simulink model "LV_Greensite"  (R2019b)
settings: Solver=ode4  StartTime=0.0  StopTime=140  FixedStep=0.01  RelTol=1e-3
values from neighbouring files (symbols this model uses):
  drywind =     [drywind.mat]
undefined symbols (not defined in the file or in its folder): GreensiteLPV, K, Qmax
libraries: cstblocks x6, simulink_extras x4, simulink x2
settings Model: SimulationMode=accelerator  Creator=Damhlaic  LastModifiedBy=mimmo
settings DataIOCC: ReturnWorkspaceOutputs=off
settings DebuggingCC: ArithmeticOperatorsInVariantConditions=warning
settings SFSimCC: CustomCodeUndefinedFunction=UseInterfaceOnly
settings RTWCC: TargetLang=C++
settings GRTTargetCC: TargetLangStandard=C++03 (ISO)  MultiInstanceERTCode=on  CodeInterfacePackaging=C++ class

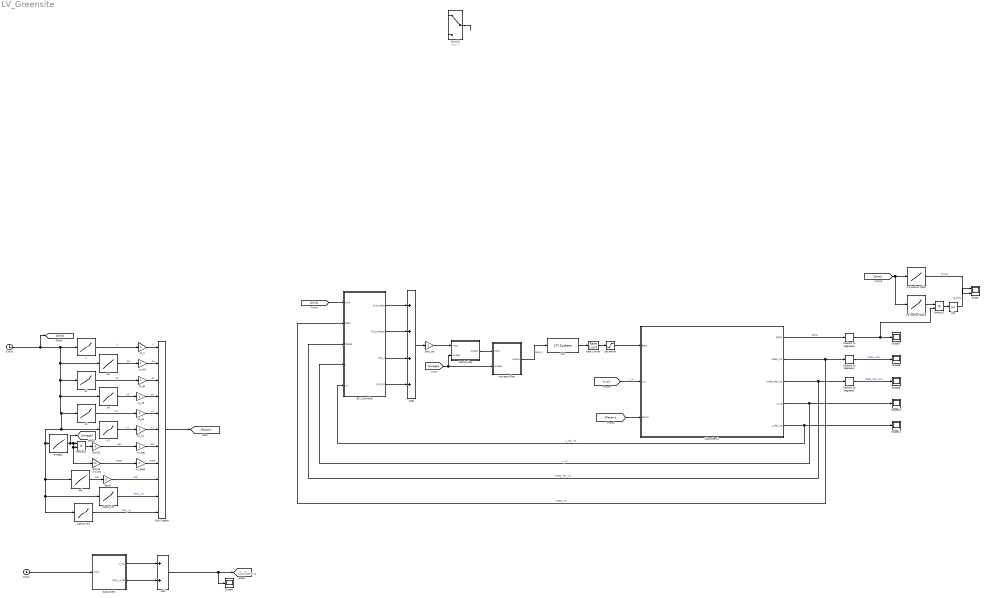
== system LV_Greensite ==
  note: 1445
      | 22360
      | 0.25
  1-D Lookup Table : Lookup_n-D  NumberOfTableDimensions=1  BreakpointsForDimension1=Qmax.time  Table=Qmax.Qalpha  InternalRulePriority=Speed  RndMeth=Simplest  InputSameDT=on
  1-D Lookup Table1 : Lookup_n-D  NumberOfTableDimensions=1  BreakpointsForDimension1=GreensiteLPV.Q.time  Table=GreensiteLPV.Q.Data  InternalRulePriority=Speed  RndMeth=Simplest  InputSameDT=on
  A6 : Lookup_n-D  NumberOfTableDimensions=1  BreakpointsForDimension1=GreensiteLPV.A6.Time  Table=GreensiteLPV.A6.Data  InternalRulePriority=Speed  RndMeth=Simplest  InputSameDT=on
  Abs : Abs
  Add : Sum
  Add1 : Sum  Inputs=++++
  BC_Controller : Subsystem
  Bus Creator : BusCreator  Inputs=11
  Clock : Clock
  Clock1 : Clock
  Gain12 : Gain  Gain=-1
  Gain13 : Gain  Gain=-2*0.005
  Gain5 : Gain  Gain=-1
  Gain_tot : Gain  Gain=-1
  K1 : Lookup_n-D  NumberOfTableDimensions=1  BreakpointsForDimension1=GreensiteLPV.K1.Time  Table=GreensiteLPV.K1.Data  InternalRulePriority=Speed  RndMeth=Simplest  InputSameDT=on
  Notch-Filter : Subsystem
  Product1 : Product
  Product2 : Product
  Radians to Degrees3 : simulink_extras/Transformations/Radians to Degrees
  Radians to Degrees4 : simulink_extras/Transformations/Radians to Degrees
  Radians to Degrees5 : simulink_extras/Transformations/Radians to Degrees
  Rate Limiter : RateLimiter  RisingSlewLimit=deg2rad(10)  FallingSlewLimit=-deg2rad(10)  SampleTimeMode=inherited
  Saturation : Saturate  UpperLimit=deg2rad(6)  LowerLimit=-deg2rad(6)
  Scope : Scope  NumInputPorts=2
  Scope{4,7..11} (6 alike) : Scope
  Subsystem : Subsystem
  Subsystem1 : Subsystem
  Switch2 : Switch  Criteria=u2 > Threshold  Threshold=7
  TVC : cstblocks/LTI System  sys=TVC_dyn  IC=[]
  V : Lookup_n-D  NumberOfTableDimensions=1  BreakpointsForDimension1=GreensiteLPV.V.Time  Table=GreensiteLPV.V.Data  InternalRulePriority=Speed  RndMeth=Simplest  InputSameDT=on
  a1 : Lookup_n-D  NumberOfTableDimensions=1  BreakpointsForDimension1=GreensiteLPV.a1.Time  Table=GreensiteLPV.a1.Data  InternalRulePriority=Speed  RndMeth=Simplest  InputSameDT=on
  a3 : Lookup_n-D  NumberOfTableDimensions=1  BreakpointsForDimension1=GreensiteLPV.a3.Time  Table=GreensiteLPV.a3.Data  InternalRulePriority=Speed  RndMeth=Simplest  InputSameDT=on
  a4 : Lookup_n-D  NumberOfTableDimensions=1  BreakpointsForDimension1=GreensiteLPV.a4.Time  Table=GreensiteLPV.a4.Data  InternalRulePriority=Speed  RndMeth=Simplest  InputSameDT=on
  aqk : Lookup_n-D  NumberOfTableDimensions=1  BreakpointsForDimension1=GreensiteLPV.aqk.Time  Table=GreensiteLPV.aqk.Data  InternalRulePriority=Speed  RndMeth=Simplest  InputSameDT=on
  low-pass filter : Subsystem
  omega1 : Lookup_n-D  NumberOfTableDimensions=1  BreakpointsForDimension1=GreensiteLPV.omega.Time  Table=GreensiteLPV.omega.Data  InternalRulePriority=Speed  RndMeth=Simplest  InputSameDT=on
  sigma_ins : Lookup_n-D  NumberOfTableDimensions=1  BreakpointsForDimension1=GreensiteLPV.sigma_ins.Time  Table=GreensiteLPV.sigma_ins.Data  InternalRulePriority=Speed  RndMeth=Simplest  InputSameDT=on
  sigma_ins1 : Lookup_n-D  NumberOfTableDimensions=1  BreakpointsForDimension1=GreensiteLPV.phi_ins.Time  Table=GreensiteLPV.phi_ins.Data  InternalRulePriority=Speed  RndMeth=Simplest  InputSameDT=on
  un_A6 : Gain
  un_K1 : Gain
  un_V : Gain
  un_a1 : Gain
  un_a3 : Gain
  un_a4 : Gain
  un_aqq : Gain
  un_aqqd : Gain
  wires:
  V/1 -> un_V/1  "V"
  A6/1 -> un_A6/1  "A6"
  a1/1 -> un_a1/1  "a1"
  a3/1 -> un_a3/1  "a3"
  a4/1 -> un_a4/1  "a4"
  Gain12/1 -> un_aqq/1  "aqq"
  Gain13/1 -> un_aqqd/1  "aqqd"
  aqk/1 -> Gain5/1  "aqk"
  sigma_ins/1 -> Bus Creator/10  "RMC_ins"
  Bus Creator/1 -> [Param]
  K1/1 -> un_K1/1  "K1"
  BC_Controller/4("Out_zd ") -> Add1/4
  BC_Controller/3(Out_z) -> Add1/3
  Radians to Degrees3/1 -> Scope9/1  "theta_dot_AAC"
  low-pass filter/1(output) -> TVC/1  "beta_c"
  Subsystem1/1(alpha) -> Radians to Degrees5/1  "alpha"
  [v_w] -> Subsystem1/2(v_w)  "v_w"
  Subsystem1/5(z_dot_ins) -> BC_Controller/5(zd), Scope11/1  "z_dot_ins"
  Subsystem1/4(z_ins) -> BC_Controller/4(z), Scope10/1  "z_ins"
  Subsystem1/3(theta_dot_ins) -> BC_Controller/3(thetad), Radians to Degrees3/1  "theta_dot_ins"
  BC_Controller/2(Out_thetad) -> Add1/2
  BC_Controller/1(Out_theta) -> Add1/1
  Add1/1 -> Gain_tot/1
  [Param] -> Subsystem1/3(param)
  Subsystem1/2(theta_ins) -> Radians to Degrees4/1, BC_Controller/2(theta)  "theta_ins"
  un_A6/1 -> Bus Creator/2  "A6"
  un_K1/1 -> Bus Creator/6  "K1"
  un_aqqd/1 -> Bus Creator/8  "aqqd"
  un_aqq/1 -> Bus Creator/7  "aqq"
  sigma_ins1/1 -> Bus Creator/11  "TMC_ins"
  Clock1/1 -> omega1/1, sigma_ins1/1, sigma_ins/1, aqk/1, K1/1, a4/1, a3/1, a1/1, A6/1, V/1, [time]
  Radians to Degrees5/1 -> Product2/2, Scope7/1
  un_V/1 -> Bus Creator/1  "V"
  un_a1/1 -> Bus Creator/3  "a1"
  un_a3/1 -> Bus Creator/4  "a3"
  un_a4/1 -> Bus Creator/5  "a4"
  Subsystem/2(noisy_wind) -> Add/2
  Subsystem/1(v_wp) -> Add/1
  Product1/1 -> Gain12/1
  [time] -> BC_Controller/1(time)
  Gain5/1 -> Bus Creator/9  "aqk"
  1-D Lookup Table1/1 -> Product2/1
  Product2/1 -> Abs/1
  1-D Lookup Table/1 -> Scope/2  "Qmax"
  [time] -> 1-D Lookup Table1/1, 1-D Lookup Table/1
  Abs/1 -> Scope/1  "Qalpha"
  Radians to Degrees4/1 -> Scope8/1  "theta_AAC"
  Add/1 -> Scope4/1, [v_w]
  Clock/1 -> Subsystem/1(clock)
  TVC/1 -> Rate Limiter/1
  Rate Limiter/1 -> Saturation/1
  Gain_tot/1 -> Notch-Filter/1(input)
  omega1/1 -> [omega], Gain13/1, Product1/2, Product1/1
  [omega] -> low-pass filter/2(omega), Notch-Filter/2(omega)
  Switch2/1 -> ?
  Saturation/1 -> Subsystem1/1(Beta)
  Notch-Filter/1(output) -> low-pass filter/1(input)

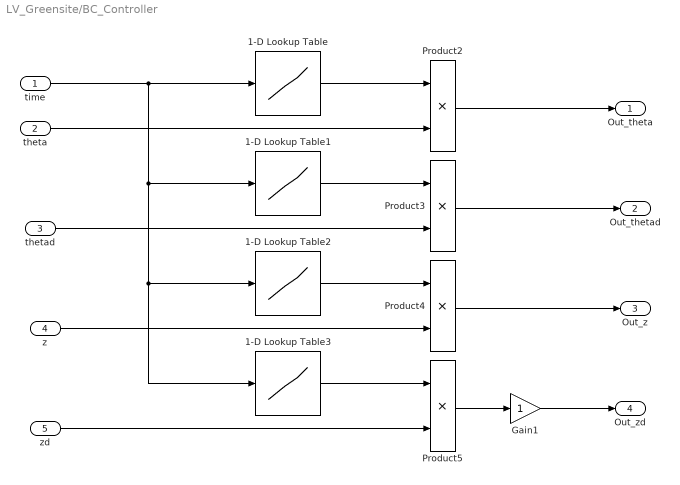
== system LV_Greensite/BC_Controller ==
  time : Inport
  theta : Inport  Port=2
  thetad : Inport  Port=3
  z : Inport  Port=4
  zd : Inport  Port=5
  1-D Lookup Table : Lookup_n-D  NumberOfTableDimensions=1  BreakpointsForDimension1=K.time  Table=K.Ktheta  InternalRulePriority=Speed  RndMeth=Simplest  InputSameDT=on
  1-D Lookup Table1 : Lookup_n-D  NumberOfTableDimensions=1  BreakpointsForDimension1=K.time  Table=K.Kthetad  InternalRulePriority=Speed  RndMeth=Simplest  InputSameDT=on
  1-D Lookup Table2 : Lookup_n-D  NumberOfTableDimensions=1  BreakpointsForDimension1=K.time  Table=K.Kz  InternalRulePriority=Speed  RndMeth=Simplest  InputSameDT=on
  1-D Lookup Table3 : Lookup_n-D  NumberOfTableDimensions=1  BreakpointsForDimension1=K.time  Table=K.Kzd  InternalRulePriority=Speed  RndMeth=Simplest  InputSameDT=on
  Gain1 : Gain
  Product{2..5} (4 alike) : Product
  Out_theta : Outport
  Out_thetad : Outport  Port=2
  Out_z : Outport  Port=3
  "Out_zd " : Outport  Port=4
  wires:
  zd/1 -> Product5/2
  1-D Lookup Table/1 -> Product2/1
  time/1 -> 1-D Lookup Table3/1, 1-D Lookup Table2/1, 1-D Lookup Table1/1, 1-D Lookup Table/1
  1-D Lookup Table3/1 -> Product5/1
  Product2/1 -> Out_theta/1
  1-D Lookup Table1/1 -> Product3/1
  1-D Lookup Table2/1 -> Product4/1
  thetad/1 -> Product3/2
  z/1 -> Product4/2
  Product3/1 -> Out_thetad/1
  theta/1 -> Product2/2
  Product5/1 -> Gain1/1
  Product4/1 -> Out_z/1
  Gain1/1 -> "Out_zd "/1

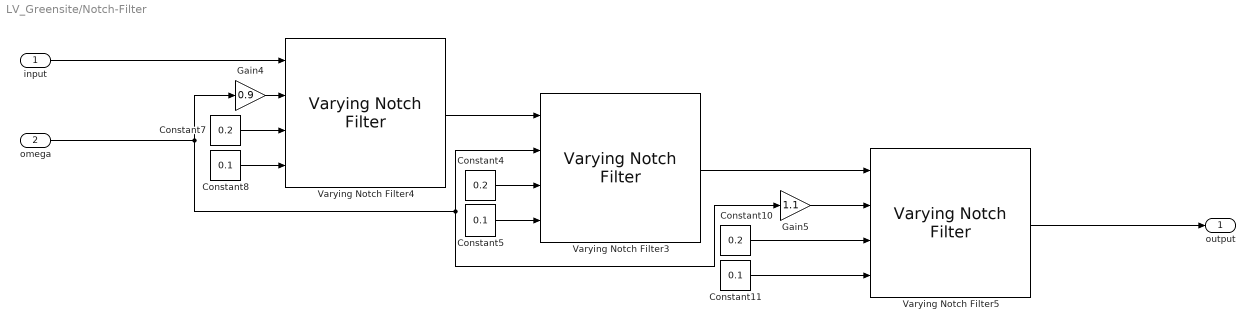
== system LV_Greensite/Notch-Filter ==
  input : Inport
  omega : Inport  Port=2
  Constant10 : Constant  Value=0.2
  Constant11 : Constant  Value=0.1
  Constant4 : Constant  Value=0.2
  Constant5 : Constant  Value=0.1
  Constant7 : Constant  Value=0.2
  Constant8 : Constant  Value=0.1
  Gain4 : Gain  Gain=0.9
  Gain5 : Gain  Gain=1.1
  Varying Notch Filter3 : cstblocks/Linear Parameter Varying/Varying Notch Filter
      settings: SourceProductName=Control System Toolbox  SourceProductBaseCode=CT
  Varying Notch Filter4 : cstblocks/Linear Parameter Varying/Varying Notch Filter
      settings: SourceProductName=Control System Toolbox  SourceProductBaseCode=CT
  Varying Notch Filter5 : cstblocks/Linear Parameter Varying/Varying Notch Filter
      settings: SourceProductName=Control System Toolbox  SourceProductBaseCode=CT
  output : Outport
  wires:
  Constant8/1 -> Varying Notch Filter4/4
  Gain5/1 -> Varying Notch Filter5/2
  Varying Notch Filter3/1 -> Varying Notch Filter5/1
  Constant11/1 -> Varying Notch Filter5/4
  Constant10/1 -> Varying Notch Filter5/3
  Gain4/1 -> Varying Notch Filter4/2
  Constant4/1 -> Varying Notch Filter3/3
  Constant7/1 -> Varying Notch Filter4/3
  Constant5/1 -> Varying Notch Filter3/4
  Varying Notch Filter4/1 -> Varying Notch Filter3/1
  input/1 -> Varying Notch Filter4/1
  Varying Notch Filter5/1 -> output/1
  omega/1 -> Gain4/1, Gain5/1, Varying Notch Filter3/2

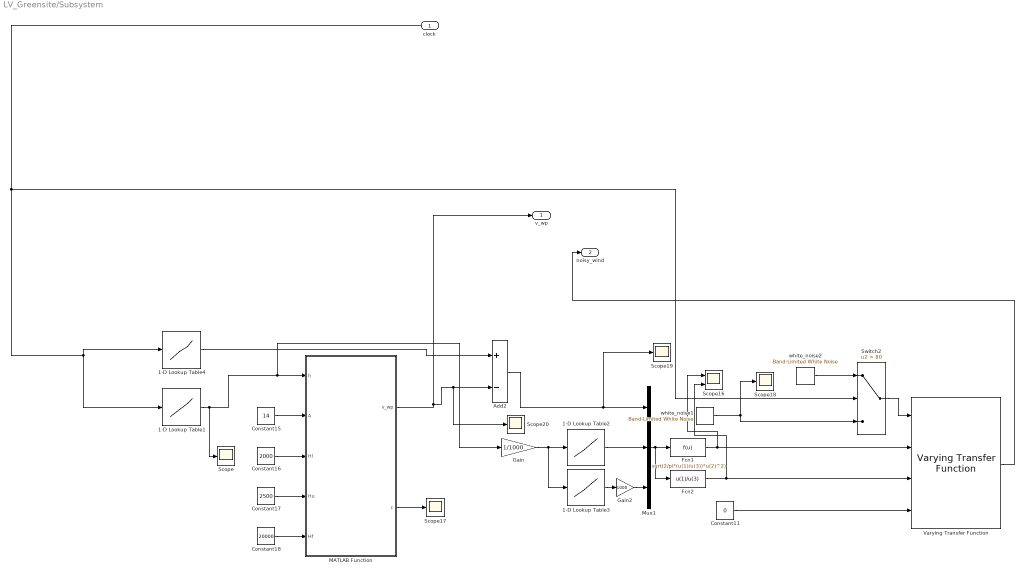
== system LV_Greensite/Subsystem ==
  clock : Inport
  1-D Lookup Table1 : Lookup_n-D  NumberOfTableDimensions=1  BreakpointsForDimension1=GreensiteLPV.h.Time  Table=GreensiteLPV.h.Data  InternalRulePriority=Speed  RndMeth=Simplest  InputSameDT=on
  1-D Lookup Table2 : Lookup_n-D  NumberOfTableDimensions=1  BreakpointsForDimension1=drywind.alt  Table=drywind.sigma.severe  InternalRulePriority=Speed  RndMeth=Simplest  InputSameDT=on
  1-D Lookup Table3 : Lookup_n-D  NumberOfTableDimensions=1  BreakpointsForDimension1=drywind.alt  Table=drywind.Lh  InternalRulePriority=Speed  RndMeth=Simplest  InputSameDT=on
  1-D Lookup Table4 : Lookup_n-D  NumberOfTableDimensions=1  BreakpointsForDimension1=GreensiteLPV.V.Time  Table=GreensiteLPV.V.Data  InternalRulePriority=Speed  RndMeth=Simplest  InputSameDT=on
  Add2 : Sum  Inputs=+-
  Constant11 : Constant  Value=0
  Constant15 : Constant  Value=14
  Constant16 : Constant  Value=2000
  Constant17 : Constant  Value=2500
  Constant18 : Constant  Value=20000
  Fcn1 : Fcn  Expr=sqrt(2/pi*(u(1)/u(3))*u(2)^2)
  Fcn2 : Fcn  Expr=u(1)/u(3)
  Gain : Gain  Gain=1/1000
  Gain2 : Gain  Gain=1000
  MATLAB Function : MATLAB Function  TreatAsAtomicUnit=on
  Mux1 : Mux  Inputs=3
  Scope{,17..20} (5 alike) : Scope
  Scope16 : Scope  NumInputPorts=2
  Switch2 : Switch  Criteria=u2 > Threshold  Threshold=80
  Varying Transfer Function : cstblocks/Linear Parameter Varying/Varying Transfer Function  N=1
      settings: SourceProductName=Control System Toolbox
  white_noise1 : simulink/Sources/Band-Limited White Noise  Cov=[1]  Ts=0.1  seed=22222
  white_noise2 : simulink/Sources/Band-Limited White Noise  Cov=[0.01]  Ts=0.1  seed=22222
  v_wp : Outport
  noisy_wind : Outport  Port=2
  wires:
  Add2/1 -> Mux1/1, Scope19/1
  1-D Lookup Table4/1 -> Add2/1
  MATLAB Function/1(v_wp) -> v_wp/1, Add2/2, Scope20/1
  Gain2/1 -> Mux1/3
  Mux1/1 -> Fcn1/1, Fcn2/1
  1-D Lookup Table1/1 -> Scope/1, MATLAB Function/1(h), Gain/1
  clock/1 -> 1-D Lookup Table1/1, 1-D Lookup Table4/1, Switch2/2
  Constant15/1 -> MATLAB Function/2(A)
  white_noise1/1 -> Switch2/3, Scope18/1
  Constant16/1 -> MATLAB Function/3(Hl)
  MATLAB Function/2(c) -> Scope17/1
  white_noise2/1 -> Switch2/1
  Switch2/1 -> Varying Transfer Function/1
  Fcn2/1 -> Varying Transfer Function/3, Scope16/2
  Constant11/1 -> Varying Transfer Function/4
  Varying Transfer Function/1 -> noisy_wind/1
  1-D Lookup Table3/1 -> Gain2/1
  Gain/1 -> 1-D Lookup Table2/1, 1-D Lookup Table3/1
  1-D Lookup Table2/1 -> Mux1/2
  Constant18/1 -> MATLAB Function/5(Hf)
  Constant17/1 -> MATLAB Function/4(Hu)
  Fcn1/1 -> Varying Transfer Function/2, Scope16/1

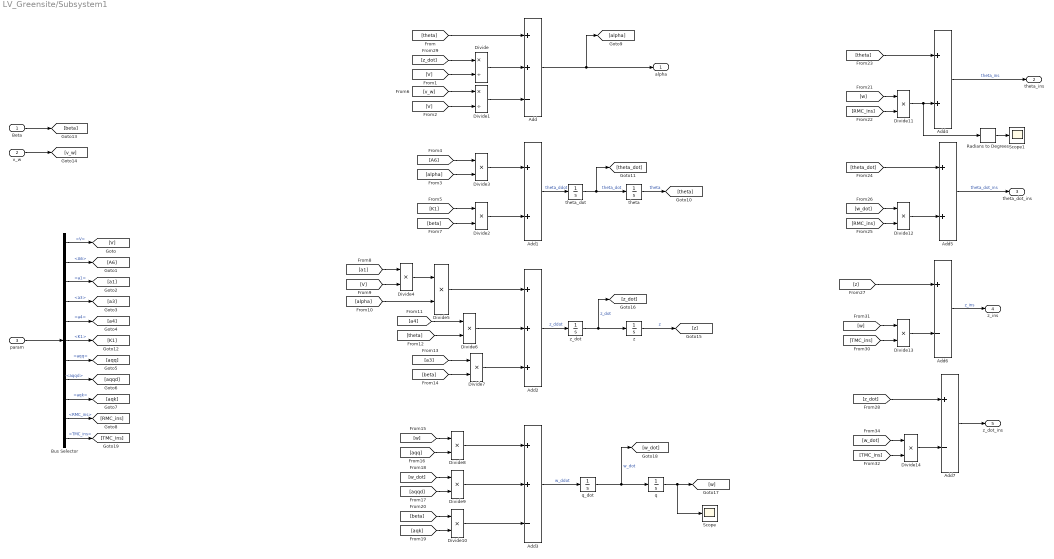
== system LV_Greensite/Subsystem1 ==
  Beta : Inport
  v_w : Inport  Port=2
  param : Inport  Port=3
  Add : Sum  Inputs=++-
  Add1 : Sum
  Add2 : Sum  Inputs=+++
  Add3 : Sum  Inputs=++-
  Add4 : Sum
  Add5 : Sum
  Add6 : Sum  Inputs=+-
  Add7 : Sum  Inputs=+-
  Bus Selector : BusSelector  OutputSignals=V,A6,a1,a3,a4,K1,aqq,aqqd,aqk,RMC_ins,TMC_ins
  Divide : Product  Inputs=*/
  Divide1 : Product  Inputs=*/
  Divide{2..14} (13 alike) : Product  Inputs=**
  Radians to Degrees : simulink_extras/Transformations/Radians to Degrees
  Scope : Scope
  Scope1 : Scope
  q : Integrator
  q_dot : Integrator
  theta : Integrator
  theta_dot : Integrator
  z : Integrator
  z_dot : Integrator
  alpha : Outport  VectorParamsAs1DForOutWhenUnconnected=off
  theta_ins : Outport  Port=2  VectorParamsAs1DForOutWhenUnconnected=off
  theta_dot_ins : Outport  Port=3  VectorParamsAs1DForOutWhenUnconnected=off
  z_ins : Outport  Port=4  VectorParamsAs1DForOutWhenUnconnected=off
  z_dot_ins : Outport  Port=5  VectorParamsAs1DForOutWhenUnconnected=off
  wires:
  [z_dot] -> Add7/1
  [TMC_ins] -> Divide14/2
  [w_dot] -> Divide14/1
  Divide14/1 -> Add7/2
  Add6/1 -> z_ins/1  "z_ins"
  [z] -> Add6/1
  [TMC_ins] -> Divide13/2
  [w] -> Divide13/1
  Divide13/1 -> Add6/2
  Bus Selector/11 -> [TMC_ins]  "<TMC_ins>"
  Divide/1 -> Add/2
  Divide11/1 -> Radians to Degrees/1, Add4/2
  [z_dot] -> Divide/1
  Add7/1 -> z_dot_ins/1
  Add5/1 -> theta_dot_ins/1  "theta_dot_ins"
  Divide12/1 -> Add5/2
  [w_dot] -> Divide12/1
  [RMC_ins] -> Divide12/2
  [theta_dot] -> Add5/1
  [theta] -> Add4/1
  [RMC_ins] -> Divide11/2
  [w] -> Divide11/1
  Add4/1 -> theta_ins/1  "theta_ins"
  [beta] -> Divide10/1
  [aqk] -> Divide10/2
  Divide10/1 -> Add3/3
  [w_dot] -> Divide9/1
  [aqqd] -> Divide9/2
  Divide9/1 -> Add3/2
  [aqq] -> Divide8/2
  Divide8/1 -> Add3/1
  [w] -> Divide8/1
  q/1 -> [w], Scope/1
  q_dot/1 -> q/1, [w_dot]  "w_dot"
  Add3/1 -> q_dot/1  "w_ddot"
  Divide7/1 -> Add2/3
  [a3] -> Divide7/1
  [beta] -> Divide7/2
  Divide6/1 -> Add2/2
  [theta] -> Divide6/2
  [a4] -> Divide6/1
  Divide5/1 -> Add2/1
  [alpha] -> Divide5/2
  Divide4/1 -> Divide5/1
  [V] -> Divide4/2
  [a1] -> Divide4/1
  z/1 -> [z]  "z"
  z_dot/1 -> z/1, [z_dot]  "z_dot"
  Add2/1 -> z_dot/1  "z_ddot"
  [beta] -> Divide2/2
  [v_w] -> Divide1/1
  v_w/1 -> [v_w]
  Beta/1 -> [beta]
  [K1] -> Divide2/1
  Bus Selector/6 -> [K1]  "<K1>"
  [A6] -> Divide3/1
  [alpha] -> Divide3/2
  Divide3/1 -> Add1/1
  Divide2/1 -> Add1/2
  [V] -> Divide1/2
  [V] -> Divide/2
  Add1/1 -> theta_dot/1  "theta_ddot"
  theta/1 -> [theta]  "theta"
  theta_dot/1 -> theta/1, [theta_dot]  "theta_dot"
  Add/1 -> alpha/1, [alpha]
  [theta] -> Add/1
  Divide1/1 -> Add/3
  Bus Selector/10 -> [RMC_ins]  "<RMC_ins>"
  Bus Selector/9 -> [aqk]  "<aqk>"
  Bus Selector/8 -> [aqqd]  "<aqqd>"
  Bus Selector/7 -> [aqq]  "<aqq>"
  Bus Selector/5 -> [a4]  "<a4>"
  Bus Selector/4 -> [a3]  "<a3>"
  Bus Selector/3 -> [a1]  "<a1>"
  Bus Selector/2 -> [A6]  "<A6>"
  Bus Selector/1 -> [V]  "<V>"
  param/1 -> Bus Selector/1
  Radians to Degrees/1 -> Scope1/1

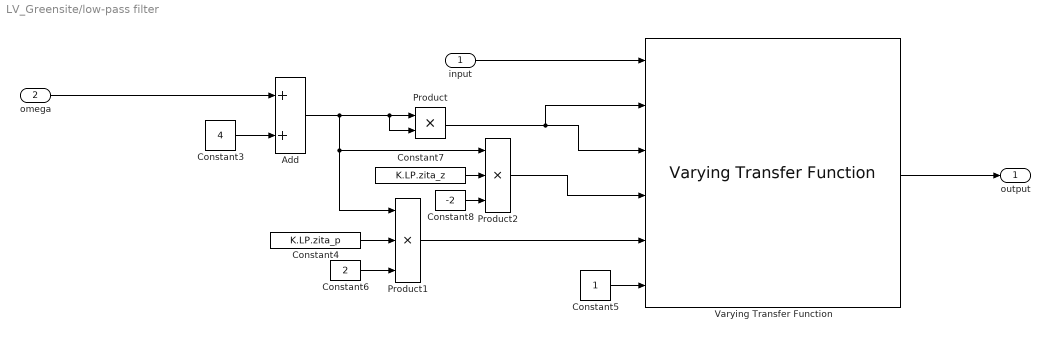
== system LV_Greensite/low-pass filter ==
  input : Inport
  omega : Inport  Port=2
  Add : Sum
  Constant3 : Constant  Value=4
  Constant4 : Constant  Value=K.LP.zita_p
  Constant5 : Constant
  Constant6 : Constant  Value=2
  Constant7 : Constant  Value=K.LP.zita_z
  Constant8 : Constant  Value=-2
  Product : Product
  Product1 : Product  Inputs=3
  Product2 : Product  Inputs=3
  Varying Transfer Function : cstblocks/Linear Parameter Varying/Varying Transfer Function  N=2
      settings: SourceProductName=Control System Toolbox
  output : Outport
  wires:
  Product1/1 -> Varying Transfer Function/5
  Product2/1 -> Varying Transfer Function/4
  Constant8/1 -> Product2/3
  Constant4/1 -> Product1/2
  Constant5/1 -> Varying Transfer Function/6
  Product/1 -> Varying Transfer Function/3, Varying Transfer Function/2
  input/1 -> Varying Transfer Function/1
  Constant3/1 -> Add/2
  Constant7/1 -> Product2/2
  Add/1 -> Product/2, Product/1, Product2/1, Product1/1
  Varying Transfer Function/1 -> output/1
  Constant6/1 -> Product1/3
  omega/1 -> Add/1

== matlab function LV_Greensite/Subsystem/MATLAB Function ==
  data: h input; v_wp output; A input; Hl input; Hu input; Hf input; c output
function [v_wp,c] = fcn(h,A,Hl,Hu,Hf)
    if h < Hl
        v_wp = 10*A*(((h/2000)^(0.9))-0.9*(h/Hl));
        c = 1;
    elseif h >= Hl & h <= Hf-Hu
        v_wp = A;
        c = 2;
    elseif h > Hf-Hu & h <=Hf
        v_wp = A/2*(1 - cos((pi/Hu)*(h-Hf)));
        c = 3;
    else 
        v_wp = 0;
        c = 4;
    end
